simulink model "PIDF_avec_xy_pour_algo"  (R2023a)
settings: Solver=VariableStepAuto  StartTime=0.0  StopTime=50  RelTol=1e-3
undefined symbols (not defined in the file or in its folder): Ca2, Ccp2, g, k, m, M
libraries: cstblocks x6
settings Model: Creator=raphb  LastModifiedBy=raphb

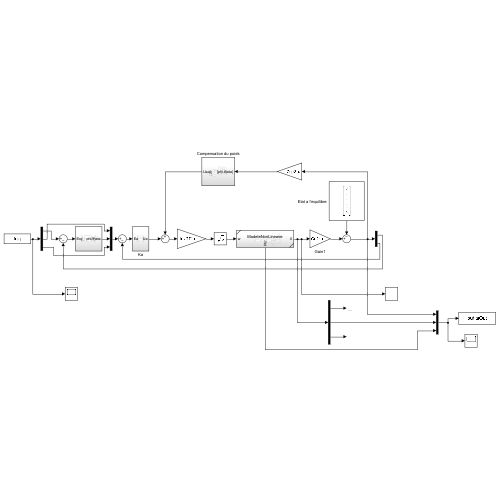
[thumbnail: Simulink's stored preview of the top-level diagram]
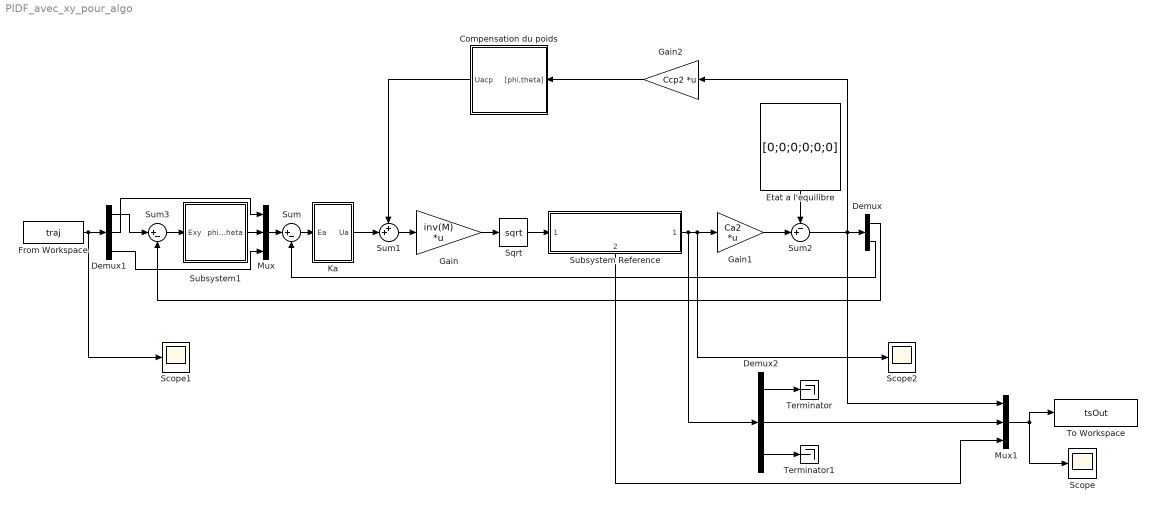
== system PIDF_avec_xy_pour_algo ==
  Compensation du poids : Subsystem
  Demux : Demux  Outputs=[2;4]
  Demux1 : Demux  Outputs=[2;1;1]
  Demux2 : Demux  Outputs=[3;3;6]
  Etat a l'equilibre : Constant  Value=[0;0;0;0;0;0]  VectorParams1D=off
  From Workspace : FromWorkspace  VariableName=traj
  Gain : Gain  Gain=inv(M)  Multiplication=Matrix(K*u)
  Gain1 : Gain  Gain=Ca2  Multiplication=Matrix(K*u)
  Gain2 : Gain  Gain=Ccp2  Multiplication=Matrix(K*u)
  Ka : Subsystem
  Mux : Mux  Inputs=[1;2;1]
  Mux1 : Mux  Inputs=3
  Scope : Scope
  Scope1 : Scope
  Scope2 : Scope
  Sqrt : Sqrt
  Subsystem Reference : Subsystem  ReferencedSubsystem=ModeleNonLineaire
      settings: PortSchema="{\"entries\":[{\"content\":{\"sides\":[{\"content\":{\"connectorIds\":[\"In1\"]},\"type\":\"ConnectorPlacement.EquallySpacedRectSide\",\"uuid\":\"2b390dc1-e46a-485f-9e73-43ae136b36b0\"},{\"content\":{\"connectorIds\":[\"Out1\"],\"side\":\"RIGHT\"},\"type\":\"ConnectorPlacement.EquallySpacedRectSide\",\"uuid\":\"93980622-cd92-4ee3-ab35-a6aca8eeb0c1\"},{\"content\":{\"side\":\"TOP\"},\"type\":\"ConnectorPlacement.EquallySpacedRectSide\",\"uuid\":\"26765f8e-c47a-4617-a80f-ce7846c0eee0\"},{\"content\":{\"connectorIds\":[\"Out2\"],\"side\":\"BOTTOM\"},\"type\":\"ConnectorPlacement.EquallySpacedRectSide\",\"uuid\":\"571f16a0-a68f-4fdf-a6eb-5beadeea1fe3\"}]},\"type\":\"ConnectorPlacement.EquallySpacedConnector\",\"uuid\":\"8911b2de-3ea1-48a0-8ef0-bc765182f137\"}],\"packageUris\":[\"http://schema.mathworks.com/mf0/Connector/R2020b\"],\"version\":\"1.0\"}"
  Subsystem1 : Subsystem
  Sum : Sum  Inputs=|+-
  Sum1 : Sum  Inputs=++|
  Sum2 : Sum  Inputs=-+|
  Sum3 : Sum  Inputs=|+-
  Terminator : Terminator
  Terminator1 : Terminator
  To Workspace : ToWorkspace  VariableName=tsOut  SaveFormat=Timeseries  SampleTime=-1
  wires:
  Compensation du poids/1(Uacp) -> Sum1/1
  Etat a l'equilibre/1 -> Sum2/1
  Gain/1 -> Sqrt/1
  Gain1/1 -> Sum2/2
  Subsystem Reference/1 -> Demux2/1, Scope2/1, Gain1/1
  Sum2/1 -> Gain2/1, Mux1/1, Demux/1
  Sum1/1 -> Gain/1
  Ka/1(Ua) -> Sum1/2
  Sqrt/1 -> Subsystem Reference/1
  Sum/1 -> Ka/1(Ea)
  Gain2/1 -> Compensation du poids/1("[phi,theta]")
  Demux/2 -> Sum/2
  Demux/1 -> Sum3/2
  Demux1/1 -> Sum3/1
  Sum3/1 -> Subsystem1/1(Exy)
  Subsystem1/1(phi/theta) -> Mux/2
  Mux/1 -> Sum/1
  Demux1/2 -> Mux/1
  Demux1/3 -> Mux/3
  From Workspace/1 -> Scope1/1, Demux1/1
  Demux2/1 -> Terminator/1
  Demux2/3 -> Terminator1/1
  Mux1/1 -> To Workspace/1, Scope/1
  Demux2/2 -> Mux1/2
  Subsystem Reference/2 -> Mux1/3

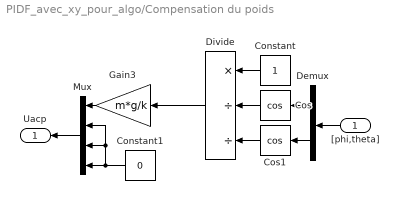
== system PIDF_avec_xy_pour_algo/Compensation du poids ==
  "[phi,theta]" : Inport
  Constant : Constant
  Constant1 : Constant  Value=0
  Cos : Trigonometry  Operator=cos
  Cos1 : Trigonometry  Operator=cos
  Demux : Demux  Outputs=2
  Divide : Product  Inputs=*//
  Gain3 : Gain  Gain=m*g/k
  Mux : Mux
  Uacp : Outport
  wires:
  Cos1/1 -> Divide/3
  Cos/1 -> Divide/2
  Demux/1 -> Cos/1
  "[phi,theta]"/1 -> Demux/1
  Demux/2 -> Cos1/1
  Constant/1 -> Divide/1
  Gain3/1 -> Mux/1
  Mux/1 -> Uacp/1
  Constant1/1 -> Mux/2, Mux/3, Mux/4
  Divide/1 -> Gain3/1

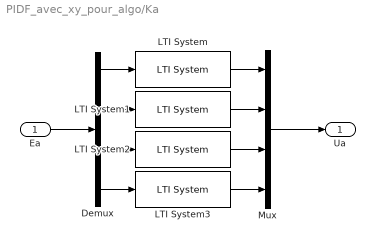
== system PIDF_avec_xy_pour_algo/Ka ==
  Ea : Inport
  Demux : Demux
  LTI System : cstblocks/LTI System  sys=Kz  IC=[]
  LTI System1 : cstblocks/LTI System  sys=Kphi  IC=[]
  LTI System2 : cstblocks/LTI System  sys=Ktheta  IC=[]
  LTI System3 : cstblocks/LTI System  sys=Kpsi  IC=[]
  Mux : Mux
  Ua : Outport
  wires:
  LTI System1/1 -> Mux/2
  Demux/4 -> LTI System3/1
  Demux/3 -> LTI System2/1
  LTI System/1 -> Mux/1
  LTI System3/1 -> Mux/4
  Ea/1 -> Demux/1
  Demux/2 -> LTI System1/1
  LTI System2/1 -> Mux/3
  Demux/1 -> LTI System/1
  Mux/1 -> Ua/1

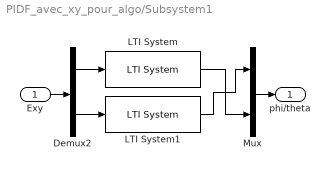
== system PIDF_avec_xy_pour_algo/Subsystem1 ==
  Exy : Inport
  Demux2 : Demux  Outputs=2
  LTI System : cstblocks/LTI System  sys=Kx  IC=[]
  LTI System1 : cstblocks/LTI System  sys=Ky  IC=[]
  Mux : Mux  Inputs=2
  phi/theta : Outport
  wires:
  LTI System/1 -> Mux/2
  LTI System1/1 -> Mux/1
  Demux2/1 -> LTI System/1
  Exy/1 -> Demux2/1
  Demux2/2 -> LTI System1/1
  Mux/1 -> phi/theta/1
